simulink model "ADRC_2RD_TEST"  (Simulink 7.6)
settings: Solver=ode45  StartTime=0.0  StopTime=50  RelTol=1e-3
libraries: ADRC x1
settings Model: Creator=Administrator  LastModifiedBy=Administrator
settings DebuggingCC: AlgebraicLoopMsg=none  ArtificialAlgebraicLoopMsg=none  SolverPrmCheckMsg=none  UnknownTsInhSupMsg=none

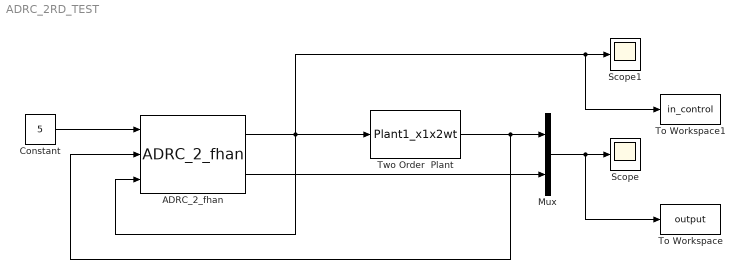
== system ADRC_2RD_TEST ==
  ADRC_2_fhan : ADRC/ADRC/ADRC_2rd/ADRC_2_fhan  SystemSampleTime=-1  h=0.01  TD=[0.1,0.01]  ESO=[100,300,1000,0.01]  NLSEF=[0.3,5,0.03]  b0=1
  Constant : Constant  Value=5
  Mux : Mux  Inputs=2
  Scope : Scope
      settings: TimeRange=20  YMin=4.9985  YMax=5.0015  DataFormat=Array
  Scope1 : Scope
      settings: TimeRange=50  YMin=0  YMax=250  DataFormat=Array
  To Workspace : ToWorkspace  VariableName=output  SampleTime=1  SaveFormat=Array
  To Workspace1 : ToWorkspace  VariableName=in_control  SampleTime=1  SaveFormat=Array
  Two Order  Plant : S-Function  FunctionName=Plant1_x1x2wt  EnableBusSupport=off
  wires:
  Constant/1 -> ADRC_2_fhan/1
  ADRC_2_fhan/1 -> ADRC_2_fhan/3, Scope1/1, To Workspace1/1, Two Order  Plant/1
  Two Order  Plant/1 -> Mux/1, ADRC_2_fhan/2
  ADRC_2_fhan/2 -> Mux/2
  Mux/1 -> To Workspace/1, Scope/1
